simulink model "pos_est_sil"  (R2024a)
settings: Solver=VariableStepAuto  StartTime=0.0  StopTime=10  FixedStep=0.001  RelTol=1e-3
settings Model: Creator=Zhenkai  LastModifiedBy=Zhenkai
settings DataIOCC: ReturnWorkspaceOutputs=off

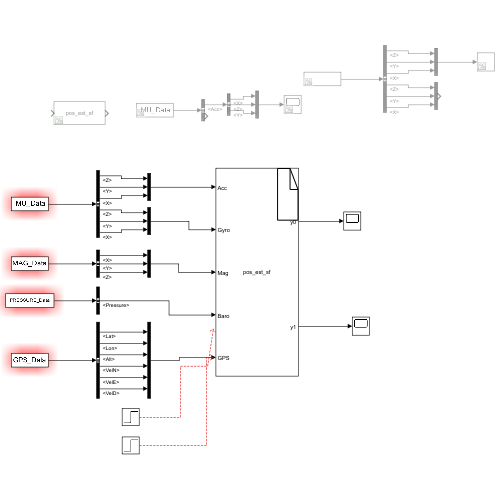
[thumbnail: Simulink's stored preview of the top-level diagram]
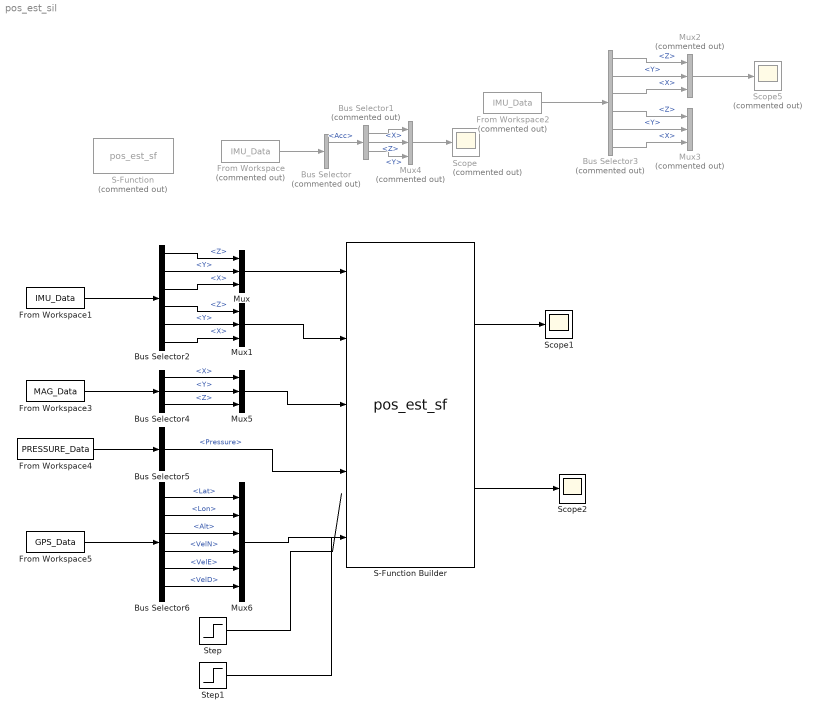
== system pos_est_sil ==
  Bus Selector : BusSelector  Commented=on  OutputSignals=Acc,Gyro
  Bus Selector1 : BusSelector  Commented=on  OutputSignals=X,Z,Y
  Bus Selector2 : BusSelector  OutputSignals=Gyro.Z,Gyro.Y,Gyro.X,Acc.Z,Acc.Y,Acc.X
  Bus Selector3 : BusSelector  Commented=on  OutputSignals=Gyro.Z,Gyro.Y,Gyro.X,Acc.Z,Acc.Y,Acc.X
  Bus Selector4 : BusSelector  OutputSignals=X,Y,Z
  Bus Selector5 : BusSelector  OutputSignals=Pressure
  Bus Selector6 : BusSelector  OutputSignals=Lat,Lon,Alt,VelN,VelE,VelD
  From Workspace : FromWorkspace  Commented=on  VariableName=IMU_Data  OutDataTypeStr=Bus: IMU_Bus  Interpolate=off  ZeroCross=off  OutputAfterFinalValue=Holding final value
  From Workspace1 : FromWorkspace  VariableName=IMU_Data  OutDataTypeStr=Bus: IMU_Bus
  From Workspace2 : FromWorkspace  Commented=on  VariableName=IMU_Data  OutDataTypeStr=Bus: IMU_Bus  Interpolate=off
  From Workspace3 : FromWorkspace  VariableName=MAG_Data  OutDataTypeStr=Bus: MAG_Bus  Interpolate=off  OutputAfterFinalValue=Holding final value
  From Workspace4 : FromWorkspace  VariableName=PRESSURE_Data  OutDataTypeStr=Bus: PRESSURE_Bus  Interpolate=off  OutputAfterFinalValue=Holding final value
  From Workspace5 : FromWorkspace  VariableName=GPS_Data  OutDataTypeStr=Bus: GPS_Bus  Interpolate=off  OutputAfterFinalValue=Holding final value
  Mux : Mux  Inputs=3
  Mux1 : Mux  Inputs=3
  Mux2 : Mux  Commented=on  Inputs=3
  Mux3 : Mux  Commented=on  Inputs=3
  Mux4 : Mux  Commented=on  Inputs=3
  Mux5 : Mux  Inputs=3
  Mux6 : Mux  Inputs=6
  S-Function : S-Function  Commented=on  FunctionName=pos_est_sf  SFunctionDeploymentMode=off  EnableBusSupport=off
  S-Function Builder : S-Function  FunctionName=pos_est_sf  SFunctionModules=pos_est_sf_wrapper.c test  SFunctionDeploymentMode=off  EnableBusSupport=off  mask(S-Function Builder){}
      mask help: Simulink:masks:SFunctionBuilder_MD
      mask init:
      | val = [[.9  0.75 0.75 1 1 .9 .9 1]',[1 1 0.75 0.75 .9 .9 1 .9]'];try , sys = get_param(gcb,'SfunBuilderFcnName');if isempty(sys), sys = get_param(gcb,'FunctionName'); end,catch, sys = get_param(gcb,'FunctionName'); end
      settings: CopyFcn=set_param(gcbh,'LinkStatus','none')  OpenFcn=sfunctionwizard(gcbh)
      mask Display:
      | plot(val(:,1),val(:,2))
      | disp(sys)
      | port_label('input',1,sprintf('%s', 'Acc'),'interpreter','tex')
      | port_label('input',2,sprintf('%s', 'Gyro'),'interpreter','tex')
      | port_label('input',3,sprintf('%s', 'Mag'),'interpreter','tex')
      | port_label('input',4,sprintf('%s', 'Baro'),'interpreter','tex')
      | port_label('input',5,sprintf('%s', 'GPS'),'interpreter','tex')
      | port_label('output',1,sprintf('%s', 'y0'),'interpreter','tex')
      | port_label('output',2,sprintf('%s', 'y1'),'interpreter','tex')
  Scope : Scope  Commented=on
  Scope1 : Scope
  Scope2 : Scope
  Scope5 : Scope  Commented=on
  Step : Step  Time=0  Before=2  After=2  SampleTime=0
  Step1 : Step  Time=0  Before=1  SampleTime=0
  wires:
  From Workspace/1 -> Bus Selector/1
  Bus Selector/1 -> Bus Selector1/1  "<Acc>"
  From Workspace1/1 -> Bus Selector2/1
  S-Function Builder/1 -> Scope1/1
  S-Function Builder/2 -> Scope2/1
  Bus Selector2/1 -> Mux/1  "<Z>"
  Bus Selector2/2 -> Mux/2  "<Y>"
  Bus Selector2/3 -> Mux/3  "<X>"
  Bus Selector2/5 -> Mux1/2  "<Y>"
  Bus Selector2/4 -> Mux1/1  "<Z>"
  Bus Selector2/6 -> Mux1/3  "<X>"
  Mux/1 -> S-Function Builder/1
  Mux1/1 -> S-Function Builder/2
  Bus Selector3/2 -> Mux2/2  "<Y>"
  Bus Selector3/5 -> Mux3/2  "<Y>"
  Bus Selector3/3 -> Mux2/3  "<X>"
  Bus Selector3/6 -> Mux3/3  "<X>"
  From Workspace2/1 -> Bus Selector3/1
  Mux2/1 -> Scope5/1
  Bus Selector3/1 -> Mux2/1  "<Z>"
  Bus Selector3/4 -> Mux3/1  "<Z>"
  Bus Selector1/1 -> Mux4/1  "<X>"
  Bus Selector1/2 -> Mux4/2  "<Z>"
  Bus Selector1/3 -> Mux4/3  "<Y>"
  Mux4/1 -> Scope/1
  From Workspace3/1 -> Bus Selector4/1
  Bus Selector4/1 -> Mux5/1  "<X>"
  Bus Selector4/2 -> Mux5/2  "<Y>"
  Bus Selector4/3 -> Mux5/3  "<Z>"
  From Workspace4/1 -> Bus Selector5/1
  From Workspace5/1 -> Bus Selector6/1
  Bus Selector6/1 -> Mux6/1  "<Lat>"
  Bus Selector6/2 -> Mux6/2  "<Lon>"
  Bus Selector6/3 -> Mux6/3  "<Alt>"
  Bus Selector6/4 -> Mux6/4  "<VelN>"
  Bus Selector6/5 -> Mux6/5  "<VelE>"
  Bus Selector6/6 -> Mux6/6  "<VelD>"
  Bus Selector5/1 -> S-Function Builder/4  "<Pressure>"
  Mux5/1 -> S-Function Builder/3
  Mux6/1 -> S-Function Builder/5
  Step/1 -> ?
  Step1/1 -> ?
